simulink model "FXLMS_simulink"  (R2019a)
settings: Solver=VariableStepAuto  StartTime=0.0  StopTime=200.0  RelTol=1e-3
values from neighbouring files (symbols this model uses):
  P = S_estw    [FXLMS.m]
  S_estw = S_estw+mu * e(k) * S_estx    [FXLMS.m]
  Sec = P    [FXLMS.m]
libraries: simulink x1, dspadpt3 x1
settings Model: Creator=CHENPOLIN  LastModifiedBy=CHENPOLIN

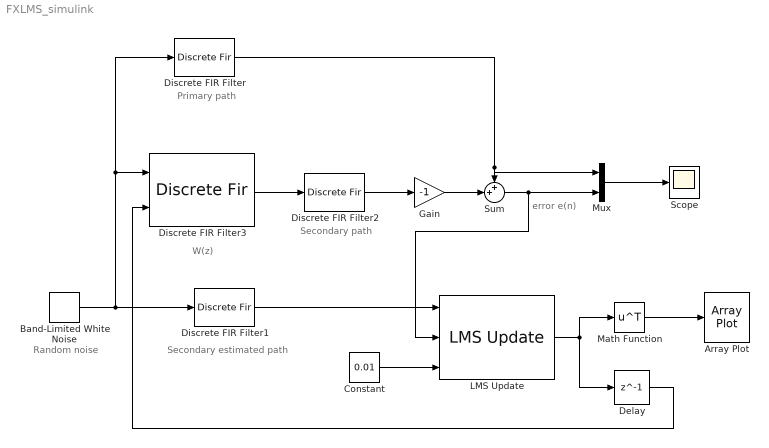
== system FXLMS_simulink ==
  note: Primary path
  note: Random noise
  note: Secondary estimated path
  note: W(z)
  note: Secondary path
  note: error e(n)
  Array Plot : ArrayPlot
  Band-Limited White Noise : simulink/Sources/Band-Limited White Noise  Cov=[0.1]  Ts=0.1  seed=[23341]
  Constant : Constant  Value=0.01
  Delay : Delay  DelayLength=1
  Discrete FIR Filter : DiscreteFir  Coefficients=P
  Discrete FIR Filter1 : DiscreteFir  Coefficients=S_estw
  Discrete FIR Filter2 : DiscreteFir  Coefficients=Sec
  Discrete FIR Filter3 : DiscreteFir  CoefSource=Input port
      settings: InputPortMap=u0,u1
  Gain : Gain  Gain=-1
  LMS Update : dspadpt3/LMS Update  Method=LMS  Length=32  StepSizeSource=Input port  StepSize=0.1  LeakageFactor=1.0  InitialConditions=0  EnableAdaptInput=off  EnableResetInput=off  SimulateUsing=Code generation
      settings: SourceProductName=DSP System Toolbox  SourceProductBaseCode=DS
  Math Function : Math  Operator=transpose  SaturateOnIntegerOverflow=on
  Mux : Mux  Inputs=2
  Scope : Scope
  Sum : Sum  Inputs=++|
  wires:
  Constant/1 -> LMS Update/3
  Discrete FIR Filter/1 -> Mux/1, Sum/1
  Discrete FIR Filter1/1 -> LMS Update/1
  Sum/1 -> Mux/2, LMS Update/2
  LMS Update/1 -> Delay/1, Math Function/1
  Math Function/1 -> Array Plot/1
  Band-Limited White Noise/1 -> Discrete FIR Filter3/1, Discrete FIR Filter/1, Discrete FIR Filter1/1
  Mux/1 -> Scope/1
  Delay/1 -> Discrete FIR Filter3/2
  Discrete FIR Filter2/1 -> Gain/1
  Discrete FIR Filter3/1 -> Discrete FIR Filter2/1
  Gain/1 -> Sum/2
